simulink model "flex_robot_flat"  (Simulink 8.5)
settings: Solver=ode45  StartTime=0.0  StopTime=100  MaxStep=1e-4  RelTol=1e-3
values from neighbouring files (symbols this model uses):
  x2a = -pi/2    (= -1.57079632679)    [params.m]
  x2e = pi/2    (= 1.57079632679)    [params.m]
settings Model: Creator=me  LastModifiedBy=cds-lue-1
settings DebuggingCC: SolverPrmCheckMsg=warning  FcnCallInpInsideContextMsg=UseLocalSettings

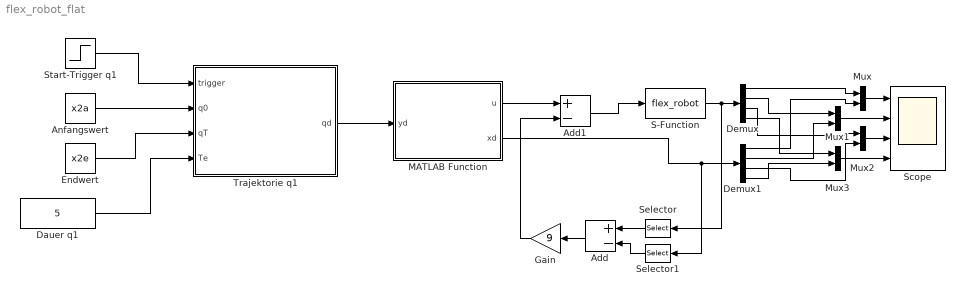
== system flex_robot_flat ==
  Add : Sum  Inputs=+-
  Add1 : Sum  Inputs=+-
  Anfangswert : Constant  Value=x2a
  Dauer q1 : Constant  Value=5
  Demux : Demux
  Demux1 : Demux
  Endwert : Constant  Value=x2e
  Gain : Gain  Gain=9
  MATLAB Function : MATLAB Function  TreatAsAtomicUnit=on
  Mux{,1..3} (4 alike) : Mux  Inputs=2
  S-Function : S-Function  FunctionName=flex_robot  Parameters=par
  Scope : Scope  NumInputPorts=4
      settings: ShowLegends=on  YMin=-2~-5~-5~-5  YMax=1.25~5~5~5
  Selector : Selector  InputPortWidth=4  Indices=2
  Selector1 : Selector  InputPortWidth=4  Indices=2
  Start-Trigger q1 : Step  SampleTime=0
  Trajektorie q1 : MATLAB Function  TreatAsAtomicUnit=on
  wires:
  Start-Trigger q1/1 -> Trajektorie q1/1(trigger)
  Anfangswert/1 -> Trajektorie q1/2(q0)
  Endwert/1 -> Trajektorie q1/3(qT)
  Dauer q1/1 -> Trajektorie q1/4(Te)
  Trajektorie q1/1(qd) -> MATLAB Function/1(yd)
  S-Function/1 -> Selector/1, Demux/1
  MATLAB Function/2(xd) -> Selector1/1, Demux1/1
  Mux/1 -> Scope/1
  Mux2/1 -> Scope/3
  Mux1/1 -> Scope/2
  Mux3/1 -> Scope/4
  Demux/1 -> Mux/1
  Demux1/1 -> Mux/2
  Demux/2 -> Mux1/1
  Demux1/2 -> Mux1/2
  Demux/3 -> Mux2/1
  Demux1/3 -> Mux2/2
  Demux/4 -> Mux3/1
  Demux1/4 -> Mux3/2
  Add/1 -> Gain/1
  Selector/1 -> Add/1
  Selector1/1 -> Add/2
  MATLAB Function/1(u) -> Add1/1
  Add1/1 -> S-Function/1
  Gain/1 -> Add1/2

== matlab function Trajektorie q1 ==
  settings: updateMethod=DISCRETE  sampleTime=1e-3
  data: trigger input double; qd output double; q0 input double; qT input double; Te input double; sysPar parameter double
function qd  = feedfw_q1(trigger,q0,qT,Te,sysPar)


beta5 = sysPar.beta5;
beta6 = sysPar.beta6;
beta7 = sysPar.beta7;
beta8 = sysPar.beta8;
beta9 = sysPar.beta9;


persistent t;

Ta=1e-3;
T=Te;
if isempty(t)
    t=0;
end
if(trigger)
    q=q0 + (qT-q0) * (beta5*(t/T)^5+beta6*(t/T)^6+beta7*(t/T)^7+beta8*(t/T)^8+beta9*(t/T)^9);
    qp=(qT - q0) * (5 * beta5 * t ^ 4 / T ^ 5 + 6 * beta6 * t ^ 5 / T ^ 6 + 7 * beta7 * t ^ 6 / T ^ 7 + 8 * beta8 * t ^ 7 / T ^ 8 + 9 * beta9 * t ^ 8 / T ^ 9);
    qpp=(qT - q0) * (20 * beta5 * t ^ 3 / T ^ 5 + 30 * beta6 * t ^ 4 / T ^ 6 + 42 * beta7 * t ^ 5 / T ^ 7 + 56 * beta8 * t ^ 6 / T ^ 8 + 72 * beta9 * t ^ 7 / T ^ 9);
    qppp=(qT - q0) * (60 * beta5 * t ^ 2 / T ^ 5 + 120 * beta6 * t ^ 3 / T ^ 6 + 210 * beta7 * t ^ 4 / T ^ 7 + 336 * beta8 * t ^ 5 / T ^ 8 + 504 * beta9 * t ^ 6 / T ^ 9); 
    qpppp=(qT - q0) * (120 * beta5 * t / T ^ 5 + 360 * beta6 * t ^ 2 / T ^ 6 + 840 * beta7 * t ^ 3 / T ^ 7 + 1680 * beta8 * t ^ 4 / T ^ 8 + 3024 * beta9 * t ^ 5 / T ^ 9);

    if t<T
        t=t+Ta;
        qd=[q;qp;qpp;qppp;qpppp];
    else
        qd=[qT;0;0;0;0];  
    end
    
else
    qd=[q0;0;0;0;0];
end

== matlab function MATLAB Function ==
  settings: updateMethod=DISCRETE  sampleTime=1e-3
  data: u output double; yd input double; par parameter double; xd output double
function [u,xd] = Vorsteuerung(yd, par)
c=10;
d1=0.5;
d2=0.5;
m=1;
g=9.81;
l=0.5;
I1=1;
I2=1;

x2 = yd(1);
x2p = yd(2);
x2pp = yd(3);
x2ppp = yd(4);
x2pppp = yd(5);
ydpppp = x2pppp;
x1 = (m * g * l * cos(x2) + x2pp * I2 + c * x2 + d2 * x2p) / c;
x3 = (-m * g * l * x2p * sin(x2) + x2ppp * I2 + c * x2p + d2 * x2pp) / c;
x4 = x2p;

u = (ydpppp + d2 / I2 ^ 2 * c * x3 - (m * g * l / I2 * cos(x2) * x4 - d2 / I2 * (-c / I2 + m * g * l / I2 * sin(x2))) * x4 - c / I2 * (-c / I1 * x1 + c / I1 * x2 - d1 / I1 * x3) - (-c / I2 + m * g * l / I2 * sin(x2) + d2 ^ 2 / I2 ^ 2) * (c / I2 * x1 - c / I2 * x2 - m * g * l / I2 * cos(x2) - d2 / I2 * x4)) / c * I2 * I1;
xd = zeros(4,1);
xd(1) = x1;
xd(2) = yd(1);
xd(3) = x3;
xd(4) = x4;
